simulink model "MCASSimulation__exp"  (R2022b)
settings: Solver=VariableStepAuto  StartTime=0.0  StopTime=350  RelTol=1e-3
model workspace (MAT data in the model file):
  ASd = 1
values from neighbouring files (symbols this model uses):
  sortedParams = table2struct(sortedT)    [RunSimulations.m]    (also in no_anomolies_run_handler.m)
libraries: slpidlib x12, simulink_extras x3
(part 3 of 4)

== matlab function MCASSimulation__exp/Human Pilot Simulator/Scripting Module/MATLAB Function Block ==
  data: JSBSim_data input; direct_to_JSBSim output; elevator_sp output; aileron_sp output; rudder_sp output; throttle_sp output; script input; horstab_sp output; script_parameters input; debug output
function [direct_to_JSBSim, elevator_sp, aileron_sp, rudder_sp, throttle_sp, horstab_sp, debug] = run(JSBSim_data, script, script_parameters)
%% Naming inputs from JSBSim
time_sec = JSBSim_data(1);
altitude_ASL_ft = JSBSim_data(2);
vert_speed_fps = JSBSim_data(3);
pitch_deg = JSBSim_data(4);
heading = JSBSim_data(5);
heading_rate_deg_sec = rad2deg(JSBSim_data(6));
roll_deg = JSBSim_data(7);
vc_kts = JSBSim_data(8);
engine_0_n1 = JSBSim_data(9);
engine_1_n1 = JSBSim_data(10);
elevator_cmd_norm = JSBSim_data(11);
stab_pos = JSBSim_data(12);
alpha = JSBSim_data(13);
mcas_is_firing = JSBSim_data(14);
mcas_cooldown_time = JSBSim_data(15);
mcas_trim_amount = JSBSim_data(16);
mcas_trim_rate = JSBSim_data(17);

mcas_duration_sec = mcas_trim_amount/mcas_trim_rate;

%% script parameters from workspace
persistent param_accel_start_spd;
persistent param_accel_end_spd;
persistent param_climb_starting_alt;
persistent param_climb_final_alt;
persistent param_desc_starting_alt;
persistent param_desc_final_alt;
persistent param_lvlturn_start_heading;
persistent param_lvlturn_turn_amount;
persistent param_climbturn_start_alt;
persistent param_climbturn_climb_amount;
persistent param_climbturn_start_heading;
persistent param_climbturn_turn_amount;
persistent param_holdpat_starting_heading;
persistent param_holdpat_leg_duration;
persistent param_takeoff_initial_climb_airspeed;
persistent param_takeoff_shallower_alt;
persistent param_takeoff_final_alt;
persistent param_takeoff_final_climb_airspeed;
persistent param_landing_desc_rate;
persistent param_landing_final_ref_airspeed;
persistent param_landing_start_alt;
persistent param_takeoffstall_target_pitch;
persistent param_takeoffstall_final_climb_airspeed;
persistent param_takeoffstall_pullup_time;
persistent param_pilot_reaction;

if isempty(param_accel_start_spd)
param_accel_start_spd = script_parameters(1);
param_accel_end_spd = script_parameters(2);
param_climb_starting_alt = script_parameters(3);
param_climb_final_alt = script_parameters(4);
param_desc_starting_alt = script_parameters(5);
param_desc_final_alt = script_parameters(6);
param_lvlturn_start_heading = script_parameters(7);
param_lvlturn_turn_amount = script_parameters(8);
param_climbturn_start_alt = script_parameters(9);
param_climbturn_climb_amount = script_parameters(10);
param_climbturn_start_heading = script_parameters(11);
param_climbturn_turn_amount = script_parameters(12);
param_holdpat_starting_heading = script_parameters(13);
param_holdpat_leg_duration = script_parameters(14);
param_takeoff_initial_climb_airspeed = script_parameters(15);
param_takeoff_shallower_alt = script_parameters(16);
param_takeoff_final_climb_airspeed = script_parameters(17);
param_takeoff_final_alt = script_parameters(18);
param_landing_desc_rate = script_parameters(19);
param_landing_final_ref_airspeed = script_parameters(20);
param_landing_start_alt = script_parameters(21);
param_takeoffstall_target_pitch = script_parameters(22);
param_takeoffstall_final_climb_airspeed = script_parameters(23);
param_takeoffstall_pullup_time = script_parameters(24);
param_pilot_reaction = script_parameters(25);
end

%% Naming controller modes
elevator_mode_off = 0;
elevator_mode_altitude = 1;
elevator_mode_vert_speed = 2;
elevator_mode_pitch = 3;
elevator_mode_airspeed = 4;
elevator_mode_direct = 5;
aileron_mode_off = 0;
aileron_mode_heading = 1;
aileron_mode_heading_rate = 2;
aileron_mode_roll = 3;
rudder_mode_off = 0;
rudder_mode_on = 1;
throttle_mode_off = 0;
throttle_mode_airspeed = 1;
throttle_mode_percent = 2;

%% Persistent variables
% Persistent variables retain their value between executions of the MATLAB function block, unlike 
% regular variables which are re-initialized each timestep of the simulation.
persistent engine_0_running;
persistent engine_1_running;
persistent landing_gear_cmd_norm;
persistent flap_cmd_norm;
persistent left_brake_cmd;
persistent right_brake_cmd;
persistent elevator_mode;
persistent ref_altitude;
persistent ref_vert_speed;
persistent ref_pitch;
persistent ref_direct;
persistent aileron_mode;
persistent ref_heading;
persistent ref_heading_rate;
persistent ref_roll;
persistent rudder_mode;
persistent ref_beta;
persistent throttle_mode;
persistent throttle_percent_norm;
persistent ref_vc;
persistent do_pilot_trim;
persistent trim_time_end;
persistent do_manual_trim;
persistent manual_trim_direction;
persistent manual_trim_time_end;
persistent lvlturn_turnto_heading;

% If a persistent variable is used only for a particular script, preface it's name with the name of the script it belongs to.
persistent level_turns_first_turn_done;

persistent climbturn_end_alt;
persistent climbturn_end_hdg;

persistent turn_then_descend_do_descent;

persistent holding_pattern_leg_timer;
persistent holding_pattern_outbound;
persistent holding_pattern_inbound;
persistent holding_pattern_inbound_heading;

persistent takeoff_step;
persistent takeoff_climb_vert_speed_fps;

persistent landing_step;

persistent takeoff_anomaly_stab_pos_start_anomaly;
persistent takeoff_anomaly_pullup_triggered;
persistent takeoff_anomaly_reacting_to_stall;
persistent takeoff_anomaly_last_mcas_turnon_time;
persistent takeoff_anomaly_retrim_start_time;

persistent takeoff_stall_pullup_triggered;
persistent takeoff_stall_reacting_to_stall;
persistent takeoff_stall_last_mcas_turnon_time;
persistent takeoff_stall_retrim_start_time;
persistent takeoff_stall_stab_pos_start_anomaly;
persistent reaction_time;


%% Scripts
switch script
    case "straight_and_level"
        if isempty(engine_0_running)
            engine_0_running = 1;
            engine_1_running = 1;
            landing_gear_cmd_norm = 0;
            flap_cmd_norm = 0;
            left_brake_cmd = 0;
            right_brake_cmd = 0;
            elevator_mode = elevator_mode_altitude;
            ref_altitude = 10000;
            ref_vert_speed = 10;
            ref_pitch = 15;
            ref_direct = 0;
            aileron_mode = aileron_mode_heading;
            ref_heading = 90;
            ref_heading_rate = 1;
            ref_roll = 15;
            rudder_mode = rudder_mode_on;
            ref_beta = 0;
            throttle_mode = throttle_mode_airspeed;
            throttle_percent_norm = 0;
            ref_vc = 240;
            do_pilot_trim = 0;  % pilot simulator will try to alleviate pressure from the elevator input
            trim_time_end = 0;
            do_manual_trim = 0;
            manual_trim_direction = 0;
            manual_trim_time_end = 0;
        end

    case "straight_and_level_accelerate"
        if isempty(engine_0_running)
            engine_0_running = 1;
            engine_1_running = 1;
            landing_gear_cmd_norm = 0;
            flap_cmd_norm = 0;
            left_brake_cmd = 0;
            right_brake_cmd = 0;
            elevator_mode = elevator_mode_altitude;
            ref_altitude = 10000;
            ref_vert_speed = 10;
            ref_pitch = 15;
            ref_direct = 0;
            aileron_mode = aileron_mode_heading;
            ref_heading = 90;
            ref_heading_rate = 1;
            ref_roll = 15;
            rudder_mode = rudder_mode_on;
            ref_beta = 0;
            throttle_mode = throttle_mode_airspeed;
            throttle_percent_norm = 0;
            ref_vc = param_accel_start_spd;
            do_pilot_trim = 0;  % pilot simulator will try to alleviate pressure from the elevator input
            trim_time_end = 0;
            do_manual_trim = 0;
            manual_trim_direction = 0;
            manual_trim_time_end = 0;
        end

        if time_sec > 15
            ref_vc = param_accel_end_spd;
        end

    case "straight_and_climb"
        if isempty(engine_0_running)
            engine_0_running = 1;
            engine_1_running = 1;
            landing_gear_cmd_norm = 0;
            flap_cmd_norm = 0;
            left_brake_cmd = 0;
            right_brake_cmd = 0;
            elevator_mode = elevator_mode_altitude;
            ref_altitude = param_climb_starting_alt;
            ref_vert_speed = 10;
            ref_pitch = 15;
            ref_direct = 0;
            aileron_mode = aileron_mode_heading;
            ref_heading = 90;
            ref_heading_rate = 1;
            ref_roll = 15;
            rudder_mode = rudder_mode_on;
            ref_beta = 0;
            throttle_mode = throttle_mode_airspeed;
            throttle_percent_norm = 0;
            ref_vc = 240;
            do_pilot_trim = 0;  % pilot simulator will try to alleviate pressure from the elevator input
            trim_time_end = 0;
            do_manual_trim = 0;
            manual_trim_direction = 0;
            manual_trim_time_end = 0;
        end

        if time_sec > 15
            ref_altitude = param_climb_final_alt;
        end

    case "straight_and_descend"
        if isempty(engine_0_running)
            engine_0_running = 1;
            engine_1_running = 1;
            landing_gear_cmd_norm = 0;
            flap_cmd_norm = 0;
            left_brake_cmd = 0;
            right_brake_cmd = 0;
            elevator_mode = elevator_mode_altitude;
            ref_altitude = param_desc_starting_alt;
            ref_vert_speed = 10;
            ref_pitch = 15;
            ref_direct = 0;
            aileron_mode = aileron_mode_heading;
            ref_heading = 90;
            ref_heading_rate = 1;
            ref_roll = 15;
            rudder_mode = rudder_mode_on;
            ref_beta = 0;
            throttle_mode = throttle_mode_airspeed;
            throttle_percent_norm = 0;
            ref_vc = 240;
            do_pilot_trim = 0;  % pilot simulator will try to alleviate pressure from the elevator input
            trim_time_end = 0;
            do_manual_trim = 0;
            manual_trim_direction = 0;
            manual_trim_time_end = 0;
        end

        if time_sec > 15
            ref_altitude = param_desc_final_alt;
        end

    case "level_turns"
        if isempty(engine_0_running)
            engine_0_running = 1;
            engine_1_running = 1;
            landing_gear_cmd_norm = 0;
            flap_cmd_norm = 0;
            left_brake_cmd = 0;
            right_brake_cmd = 0;
            elevator_mode = elevator_mode_altitude;
            ref_altitude = 10000;
            ref_vert_speed = 10;
            ref_pitch = 15;
            ref_direct = 0;
            aileron_mode = aileron_mode_heading;
            ref_heading = param_lvlturn_start_heading;
            ref_heading_rate = 1;
            ref_roll = 15;
            rudder_mode = rudder_mode_on;
            ref_beta = 0;
            throttle_mode = throttle_mode_airspeed;
            throttle_percent_norm = 0;
            ref_vc = 240;
            do_pilot_trim = 0;  % pilot simulator will try to alleviate pressure from the elevator input
            trim_time_end = 0;
            do_manual_trim = 0;
            manual_trim_direction = 0;
            manual_trim_time_end = 0;
        end
        
        if isempty(level_turns_first_turn_done) 
            level_turns_first_turn_done = 0;
            lvlturn_turnto_heading = param_lvlturn_start_heading + param_lvlturn_turn_amount;
        end

        if time_sec > 15 && ~level_turns_first_turn_done
            ref_heading = lvlturn_turnto_heading;
        end
        if heading > (lvlturn_turnto_heading-0.5) && heading < (lvlturn_turnto_heading+0.5)
            level_turns_first_turn_done = 1;
            ref_heading = param_lvlturn_start_heading;
        end

    case "climb_and_turn"
        if isempty(engine_0_running)
            engine_0_running = 1;
            engine_1_running = 1;
            landing_gear_cmd_norm = 0;
            flap_cmd_norm = 0;
            left_brake_cmd = 0;
            right_brake_cmd = 0;
            elevator_mode = elevator_mode_altitude;
            ref_altitude = param_climbturn_start_alt;
            ref_vert_speed = 10;
            ref_pitch = 15;
            ref_direct = 0;
            aileron_mode = aileron_mode_heading;
            ref_heading = param_climbturn_start_heading;
            ref_heading_rate = 1;
            ref_roll = 15;
            rudder_mode = rudder_mode_on;
            ref_beta = 0;
            throttle_mode = throttle_mode_airspeed;
            throttle_percent_norm = 0;
            ref_vc = 240;
            do_pilot_trim = 0;  % pilot simulator will try to alleviate pressure from the elevator input
            trim_time_end = 0;
            do_manual_trim = 0;
            manual_trim_direction = 0;
            manual_trim_time_end = 0;
        end
        if isempty(climbturn_end_alt)
            climbturn_end_alt = param_climbturn_start_alt + param_climbturn_climb_amount;
            climbturn_end_hdg = param_climbturn_start_heading + param_climbturn_turn_amount;
        end

        if time_sec > 15
            ref_altitude = climbturn_end_alt;
            ref_heading = climbturn_end_hdg;
        end

    case "descend_and_turn"
        if isempty(engine_0_running)
            engine_0_running = 1;
            engine_1_running = 1;
            landing_gear_cmd_norm = 0;
            flap_cmd_norm = 0;
            left_brake_cmd = 0;
            right_brake_cmd = 0;
            elevator_mode = elevator_mode_altitude;
            ref_altitude = 15000;
            ref_vert_speed = 10;
            ref_pitch = 15;
            ref_direct = 0;
            aileron_mode = aileron_mode_heading;
            ref_heading = 180;
            ref_heading_rate = 1;
            ref_roll = 15;
            rudder_mode = rudder_mode_on;
            ref_beta = 0;
            throttle_mode = throttle_mode_airspeed;
            throttle_percent_norm = 0;
            ref_vc = 240;
            do_pilot_trim = 0;  % pilot simulator will try to alleviate pressure from the elevator input
            trim_time_end = 0;
            do_manual_trim = 0;
            manual_trim_direction = 0;
            manual_trim_time_end = 0;
        end

        if time_sec > 15
            ref_altitude = 10000;
            ref_heading = 90;
        end

    case "turn_then_descend"
        if isempty(engine_0_running)
            engine_0_running = 1;
            engine_1_running = 1;
            landing_gear_cmd_norm = 0;
            flap_cmd_norm = 0;
            left_brake_cmd = 0;
            right_brake_cmd = 0;
            elevator_mode = elevator_mode_altitude;
            ref_altitude = 15000;
            ref_vert_speed = 10;
            ref_pitch = 15;
            ref_direct = 0;
            aileron_mode = aileron_mode_heading;
            ref_heading = 90;
            ref_heading_rate = 1;
            ref_roll = 15;
            rudder_mode = rudder_mode_on;
            ref_beta = 0;
            throttle_mode = throttle_mode_airspeed;
            throttle_percent_norm = 0;
            ref_vc = 240;
            do_pilot_trim = 0;  % pilot simulator will try to alleviate pressure from the elevator input
            trim_time_end = 0;
            do_manual_trim = 0;
            manual_trim_direction = 0;
            manual_trim_time_end = 0;
        end
        if isempty(turn_then_descend_do_descent)
            turn_then_descend_do_descent = 0;
        end

        if heading > 89.5 && heading < 90.5
            turn_then_descend_do_descent = 1;
        end

        if turn_then_descend_do_descent == 1
            ref_altitude = 12000;
        end

    case "holding_pattern"
        if isempty(engine_0_running)
            engine_0_running = 1;
            engine_1_running = 1;
            landing_gear_cmd_norm = 0;
            flap_cmd_norm = 0;
            left_brake_cmd = 0;
            right_brake_cmd = 0;
            elevator_mode = elevator_mode_altitude;
            ref_altitude = 10000;
            ref_vert_speed = 10;
            ref_pitch = 15;
            ref_direct = 0;
            aileron_mode = aileron_mode_heading;
            ref_heading = param_holdpat_starting_heading;
            ref_heading_rate = 1;
            ref_roll = -30; % negative = towards pilot's right
            rudder_mode = rudder_mode_on;
            ref_beta = 0;
            throttle_mode = throttle_mode_airspeed;
            throttle_percent_norm = 0;
            ref_vc = 240;
            do_pilot_trim = 0;  % pilot simulator will try to alleviate pressure from the elevator input
            trim_time_end = 0;
            do_manual_trim = 0;
            manual_trim_direction = 0;
            manual_trim_time_end = 0;
        end
        if isempty(holding_pattern_leg_timer)
            holding_pattern_leg_timer = 0;
        end
        if isempty(holding_pattern_outbound)
            holding_pattern_outbound = 0;
        end
        if isempty(holding_pattern_inbound)
            holding_pattern_inbound = 0;
        end
        if isempty(holding_pattern_inbound_heading)
            holding_pattern_inbound_heading = mod(param_holdpat_starting_heading + 180, 360);
        end

        % at heading 90
        % start timer
        if heading > (param_holdpat_starting_heading-0.5) && heading < (param_holdpat_starting_heading+0.5) && ~holding_pattern_outbound
            holding_pattern_leg_timer = time_sec;
            holding_pattern_outbound = 1;
        end

        % when timer reaches 60 seconds
        % switch aileron mode to bank 30
        if (time_sec - holding_pattern_leg_timer > param_holdpat_leg_duration) && holding_pattern_outbound
            aileron_mode = aileron_mode_roll;
        end

        % at heading 0
        % switch aileron mode to heading 270
        if heading > mod(param_holdpat_starting_heading-90.5, 360) && heading < mod(param_holdpat_starting_heading-89.5, 360) && holding_pattern_outbound
            aileron_mode = aileron_mode_heading;
            ref_heading = holding_pattern_inbound_heading;
            holding_pattern_outbound = 0;
        end

        % at heading 270
        % start timer
        if heading > (holding_pattern_inbound_heading-0.5) && heading < (holding_pattern_inbound_heading+0.5) && ~holding_pattern_inbound
            holding_pattern_leg_timer = time_sec;
            holding_pattern_inbound = 1;
        end

        % when timer reaches 60 seconds
        % switch aileron mode to bank 30
        if (time_sec - holding_pattern_leg_timer > param_holdpat_leg_duration) && holding_pattern_inbound
            aileron_mode = aileron_mode_roll;
        end

        % at heading 180
        % switch aileron mode to heading 90
        if heading > mod(param_holdpat_starting_heading+89.5, 360) && heading < mod(param_holdpat_starting_heading+90.5, 360) && holding_pattern_inbound
            aileron_mode = aileron_mode_heading;
            ref_heading = param_holdpat_starting_heading;
            holding_pattern_inbound = 0;
        end

    case "takeoff"
        if isempty(engine_0_running)
            engine_0_running = 1;
            engine_1_running = 1;
            landing_gear_cmd_norm = 1;
            flap_cmd_norm = 0.375;
            left_brake_cmd = 0;
            right_brake_cmd = 0;
            elevator_mode = elevator_mode_off;
            ref_altitude = 1000;
            ref_vert_speed = 10;
            ref_pitch = 30;
            ref_direct = 0;
            aileron_mode = aileron_mode_heading;
            ref_heading = 90;
            ref_heading_rate = 1;
            ref_roll = 15;
            rudder_mode = rudder_mode_on;
            ref_beta = 0;
            throttle_mode = throttle_mode_percent;
            throttle_percent_norm = 0;
            ref_vc = 0;
            do_pilot_trim = 0;  % pilot simulator will try to alleviate pressure from the elevator input
            trim_time_end = 0;
            do_manual_trim = 0;
            manual_trim_direction = 1;
            manual_trim_time_end = 0;
        end
        if isempty(takeoff_step)
            takeoff_step = 0;   % for ensuring each step only executes once
            takeoff_climb_vert_speed_fps = 0;
        end

        if time_sec < trim_time_end
            do_pilot_trim = 1;
        end
        if time_sec > trim_time_end
            do_pilot_trim = 0;
        end

        if time_sec > 15 && takeoff_step == 0
            throttle_percent_norm = 0.5;
            takeoff_step = takeoff_step + 1;
        end

        if engine_0_n1 > 40 && engine_1_n1 > 40 && takeoff_step == 1
            throttle_percent_norm = 0.95;
            takeoff_step = takeoff_step + 1;
        end

        if vc_kts > 150 && takeoff_step == 2    % Plane will not lift off until about 150
            elevator_mode = elevator_mode_pitch;
            ref_pitch = 10;
            takeoff_step = takeoff_step + 1;
        end

        if vc_kts > (param_takeoff_initial_climb_airspeed-10) && altitude_ASL_ft > 50 && takeoff_step == 3
            landing_gear_cmd_norm = 0;
            elevator_mode = elevator_mode_airspeed;
            ref_vc = param_takeoff_initial_climb_airspeed;
            takeoff_step = takeoff_step + 1;
        end

        if altitude_ASL_ft > 500 && takeoff_step == 4
%             trim_time_end = time_sec + 5;
            takeoff_step = takeoff_step + 1;
        end

        % 1600 ft chosen to match Lion Air crash data
        if altitude_ASL_ft > param_takeoff_shallower_alt && takeoff_step == 5
            takeoff_climb_vert_speed_fps = vert_speed_fps;
            elevator_mode = elevator_mode_vert_speed;
            ref_vert_speed = takeoff_climb_vert_speed_fps / 2;

            throttle_mode = throttle_mode_airspeed;
            ref_vc = param_takeoff_final_climb_airspeed;

            takeoff_step = takeoff_step + 1;
        end

        if altitude_ASL_ft > (param_takeoff_shallower_alt+500) && takeoff_step == 6
            trim_time_end = time_sec + 5;
            takeoff_step = takeoff_step + 1;
        end

        if vc_kts > 190
            flap_cmd_norm = 0.125;
        end

        if vc_kts > 210
            flap_cmd_norm = 0;
        end

        if altitude_ASL_ft > (param_takeoff_final_alt-500) && takeoff_step == 7     % at this point, takeoff and initial climb procedures are over, and we climb to cruise at arbitrary 15k feet.
            elevator_mode = elevator_mode_altitude;
            ref_altitude = param_takeoff_final_alt;
            takeoff_step = takeoff_step + 1;
        end

    case "landing"
       if isempty(engine_0_running)
            engine_0_running = 1;
            engine_1_running = 1;
            landing_gear_cmd_norm = 1;
            flap_cmd_norm = 0.375;
            left_brake_cmd = 0;
            right_brake_cmd = 0;
            elevator_mode = elevator_mode_altitude;
            ref_altitude = param_landing_start_alt;
            ref_vert_speed = param_landing_desc_rate;    % -700 fpm = -11.67 fps
            ref_pitch = 30;
            ref_direct = 0;
            aileron_mode = aileron_mode_heading;
            ref_heading = 90;
            ref_heading_rate = 1;
            ref_roll = 15;
            rudder_mode = rudder_mode_on;
            ref_beta = 0;
            throttle_mode = throttle_mode_airspeed;
            throttle_percent_norm = 0;
            ref_vc = 200;
            do_pilot_trim = 0;  % pilot simulator will try to alleviate pressure from the elevator input
            trim_time_end = 0;
            do_manual_trim = 0;
            manual_trim_direction = 0;
            manual_trim_time_end = 0;
       end
       if isempty(landing_step)
            landing_step = 0;   % for ensuring each step only executes once
       end

       if time_sec > 15 && landing_step == 0 
            ref_vc = param_landing_final_ref_airspeed;
            landing_step = landing_step + 1;
       end

       if vc_kts < 170 && landing_step == 1
            flap_cmd_norm = 0.5;
            landing_step = landing_step + 1;
       end

       if vc_kts < (param_landing_final_ref_airspeed+15) && landing_step == 2
           elevator_mode = elevator_mode_vert_speed;
           landing_step = landing_step + 1;
       end

       if vc_kts < 150 && landing_step == 3
           flap_cmd_norm = 0.625;
           landing_step = landing_step + 1;
       end

       if vc_kts < 140 && landing_step == 4
           flap_cmd_norm = 0.875;
           landing_step = landing_step + 1;
       end

    case "takeoff_stall_perfect_pilot"
       if isempty(engine_0_running)
            engine_0_running = 1;
            engine_1_running = 1;
            landing_gear_cmd_norm = 1;
            flap_cmd_norm = 0.375;
            left_brake_cmd = 0;
            right_brake_cmd = 0;
            elevator_mode = elevator_mode_off;
            ref_altitude = 1000;
            ref_vert_speed = 10;
            ref_pitch = 30;
            ref_direct = 0;
            aileron_mode = aileron_mode_heading;
            ref_heading = 90;
            ref_heading_rate = 1;
            ref_roll = 15;
            rudder_mode = rudder_mode_on;
            ref_beta = 0;
            throttle_mode = throttle_mode_percent;
            throttle_percent_norm = 0;
            ref_vc = 0;
            do_pilot_trim = 0;  % pilot simulator will try to alleviate pressure from the elevator input
            trim_time_end = 0;
            do_manual_trim = 0;
            manual_trim_direction = 0;
            manual_trim_time_end = 0;
        end
        if isempty(takeoff_step)
            takeoff_step = 0;   % for ensuring each step only executes once
            takeoff_climb_vert_speed_fps = 0;
        end
        if isempty(takeoff_stall_pullup_triggered)
            takeoff_stall_pullup_triggered = 0;
        end

        if time_sec > param_takeoffstall_pullup_time && ~takeoff_stall_pullup_triggered
            takeoff_stall_pullup_triggered = 1;
            elevator_mode = elevator_mode_pitch;
            ref_pitch = param_takeoffstall_target_pitch;
        end

        if alpha > 12 && takeoff_stall_pullup_triggered && takeoff_step ~= -1
            % this is where pilot begins to take action for stall
            % avoidance and recovery
            takeoff_step = -1;
            elevator_mode = elevator_mode_direct;   % aggressive nose-down to avoid immediate stall
            ref_direct = 0.6;
            throttle_mode = throttle_mode_percent;
            throttle_percent_norm = 1;
        end

        if pitch_deg < 5 && takeoff_step == -1
            takeoff_step = -2;
            elevator_mode = elevator_mode_pitch;
            ref_pitch = -4;
        end

        if vc_kts > 220 && takeoff_step == -2
            takeoff_step = 5;

            elevator_mode = elevator_mode_vert_speed;
            ref_vert_speed = takeoff_climb_vert_speed_fps / 2;  % doesn't exist if stall is initiated BEFORE the 'shallowing' step of takeoff (step 4)

            throttle_mode = throttle_mode_airspeed;
            ref_vc = param_takeoffstall_final_climb_airspeed;
        end

        if time_sec > 15 && takeoff_step == 0
            throttle_percent_norm = 0.5;
            takeoff_step = takeoff_step + 1;
        end

        if engine_0_n1 > 40 && engine_1_n1 > 40 && takeoff_step == 1
            throttle_percent_norm = 0.95;
            takeoff_step = takeoff_step + 1;
        end

        if vc_kts > 150 && takeoff_step == 2
            elevator_mode = elevator_mode_pitch;
            ref_pitch = 10;
            takeoff_step = takeoff_step + 1;
        end

        if vc_kts > 170 && altitude_ASL_ft > 50 && takeoff_step == 3
            landing_gear_cmd_norm = 0;
            elevator_mode = elevator_mode_airspeed;
            ref_vc = 170;
            takeoff_step = takeoff_step + 1;
        end

        % 1600 ft chosen to match Lion Air crash data
        if altitude_ASL_ft > 1600 && takeoff_step == 4
            takeoff_climb_vert_speed_fps = vert_speed_fps;
            elevator_mode = elevator_mode_vert_speed;
            ref_vert_speed = takeoff_climb_vert_speed_fps / 2;

            throttle_mode = throttle_mode_airspeed;
            ref_vc = param_takeoffstall_final_climb_airspeed;

            takeoff_step = takeoff_step + 1;
        end

        if vc_kts > 190 && takeoff_step == 5
            flap_cmd_norm = 0.125;
            takeoff_step = takeoff_step + 1;
        end

        if vc_kts > 210 && takeoff_step == 6
            flap_cmd_norm = 0;
            takeoff_step = takeoff_step + 1;
        end

    case "takeoff_stall_pilot_reaction_delay"
       if isempty(engine_0_running)
            engine_0_running = 1;
            engine_1_running = 1;
            landing_gear_cmd_norm = 1;
            flap_cmd_norm = 0.375;
            left_brake_cmd = 0;
            right_brake_cmd = 0;
            elevator_mode = elevator_mode_off;
            ref_altitude = 1000;
            ref_vert_speed = 10;
            ref_pitch = 30;
            ref_direct = 0;
            aileron_mode = aileron_mode_heading;
            ref_heading = 90;
            ref_heading_rate = 1;
            ref_roll = 15;
            rudder_mode = rudder_mode_on;
            ref_beta = 0;
            throttle_mode = throttle_mode_percent;
            throttle_percent_norm = 0;
            ref_vc = 0;
            do_pilot_trim = 0;  % pilot simulator will try to alleviate pressure from the elevator input
            trim_time_end = 0;
            do_manual_trim = 0;
            manual_trim_direction = 0;
            manual_trim_time_end = 0;
        end
        if isempty(takeoff_step)
            takeoff_step = 0;   % for ensuring each step only executes once
            takeoff_climb_vert_speed_fps = 0;
        end
        if isempty(takeoff_stall_pullup_triggered)
            takeoff_stall_pullup_triggered = 0;
        end
        if isempty(takeoff_stall_reacting_to_stall)
            takeoff_stall_reacting_to_stall = 0;
        end
        if isempty(takeoff_stall_last_mcas_turnon_time)
            takeoff_stall_last_mcas_turnon_time = -999;  % setting to 0 causes issues at start
        end
        if isempty(takeoff_stall_retrim_start_time)
            takeoff_stall_retrim_start_time = -999;  % setting to 0 causes issues at start
        end
        if isempty(takeoff_stall_stab_pos_start_anomaly)
            takeoff_stall_stab_pos_start_anomaly = 0;
        end

        if time_sec > takeoff_stall_retrim_start_time && time_sec < trim_time_end
            do_pilot_trim = 1;
        end
        if time_sec > trim_time_end
            do_pilot_trim = 0;
        end

        if mcas_is_firing && (time_sec-takeoff_stall_last_mcas_turnon_time) > mcas_duration_sec
            takeoff_stall_last_mcas_turnon_time = time_sec;
        end

        % stop trimming if MCAS fires (trim wheel is yanked from pilot)
        if (time_sec-takeoff_stall_last_mcas_turnon_time) > 0 && (time_sec-takeoff_stall_last_mcas_turnon_time) < 1
            trim_time_end = 0;
        end
        
        if time_sec > param_takeoffstall_pullup_time && ~takeoff_stall_pullup_triggered
            takeoff_stall_pullup_triggered = 1;
            elevator_mode = elevator_mode_pitch;
            ref_pitch = param_takeoffstall_target_pitch;
        end

        % these cause additional stall maneuvers
        %if time_sec > 200 && time_sec < 201
        %    takeoff_stall_pullup_triggered = 0;
        %end
        %if time_sec > 300 && time_sec < 301
        %    takeoff_stall_pullup_triggered = 0;
        %end

        % If AoA<10 when MCAS triggers, fight against MCAS and trim.
        % This is the case where MCAS is 'errant'.
        if (time_sec-takeoff_stall_last_mcas_turnon_time) > 0 && (time_sec-takeoff_stall_last_mcas_turnon_time) < 0.1
            takeoff_stall_retrim_start_time = time_sec + param_pilot_reaction + mcas_duration_sec;
        end

        if (time_sec-takeoff_stall_retrim_start_time) > 0 && (time_sec-takeoff_stall_retrim_start_time) < 0.1 && ~takeoff_stall_reacting_to_stall
            trim_time_end = time_sec + 2.5/(3.5/18);
        end

        % If AoA>10 when MCAS triggers, do stall recovery after reaction delay.
        % This is the case where MCAS is 'correct'.
        if (time_sec-takeoff_stall_last_mcas_turnon_time) > param_pilot_reaction && (time_sec-takeoff_stall_last_mcas_turnon_time) < param_pilot_reaction+0.1 && ~takeoff_stall_reacting_to_stall && alpha > 10
            takeoff_step = -1;
            takeoff_stall_reacting_to_stall = 1;
            elevator_mode = elevator_mode_direct;   % aggressive nose-down to avoid immediate stall
            ref_direct = 0.6;
            throttle_mode = throttle_mode_percent;
            throttle_percent_norm = 1;
        end

        if pitch_deg < 5 && takeoff_step == -1
            takeoff_step = -2;
            elevator_mode = elevator_mode_pitch;
            ref_pitch = -10;
        end
        
        % resume normal flight
        if vc_kts > 220 && takeoff_step == -2 
            takeoff_step = 5;
            takeoff_stall_reacting_to_stall = 0;
            elevator_mode = elevator_mode_vert_speed;
            ref_vert_speed = takeoff_climb_vert_speed_fps / 2;  % doesn't exist if stall is initiated BEFORE the 'shallowing' step of takeoff (step 4)
            throttle_mode = throttle_mode_airspeed;
            ref_vc = param_takeoffstall_final_climb_airspeed;
            trim_time_end = time_sec + mcas_cooldown_time;
        end

        if time_sec > 15 && takeoff_step == 0
            throttle_percent_norm = 0.5;
            takeoff_step = takeoff_step + 1;
        end

        if engine_0_n1 > 40 && engine_1_n1 > 40 && takeoff_step == 1
            throttle_percent_norm = 0.95;
            takeoff_step = takeoff_step + 1;
        end

        if vc_kts > 150 && takeoff_step == 2
            elevator_mode = elevator_mode_pitch;
            ref_pitch = 10;
            takeoff_step = takeoff_step + 1;
        end

        if vc_kts > 170 && altitude_ASL_ft > 50 && takeoff_step == 3
            landing_gear_cmd_norm = 0;
            elevator_mode = elevator_mode_airspeed;
            ref_vc = 170;
            takeoff_step = takeoff_step + 1;
        end

        % 1600 ft chosen to match Lion Air crash data
        if altitude_ASL_ft > 1600 && takeoff_step == 4
            takeoff_climb_vert_speed_fps = vert_speed_fps;
            elevator_mode = elevator_mode_vert_speed;
            ref_vert_speed = takeoff_climb_vert_speed_fps / 2;

            throttle_mode = throttle_mode_airspeed;
            ref_vc = param_takeoffstall_final_climb_airspeed;

            takeoff_step = takeoff_step + 1;
        end

        if vc_kts > 190 && takeoff_step == 5
            flap_cmd_norm = 0.125;
            takeoff_step = takeoff_step + 1;
        end

        if vc_kts > 210 && takeoff_step == 6
            flap_cmd_norm = 0;
            takeoff_step = takeoff_step + 1;
        end

        if (time_sec-takeoff_stall_retrim_start_time) > 0 && (time_sec-takeoff_stall_retrim_start_time) < 0.1 && takeoff_step == 7
            elevator_mode = elevator_mode_direct;
            ref_direct = elevator_cmd_norm;
            takeoff_stall_stab_pos_start_anomaly = stab_pos;
            
            takeoff_step = takeoff_step + 1;
        end

        if (time_sec-takeoff_stall_retrim_start_time) > param_pilot_reaction && (time_sec-takeoff_stall_retrim_start_time) < param_pilot_reaction+0.1 && takeoff_step == 8

            if takeoff_stall_stab_pos_start_anomaly ~= stab_pos  
                elevator_mode = elevator_mode_direct;
                ref_direct = -0.1;
            else
                elevator_mode = elevator_mode_vert_speed;
                ref_vert_speed = takeoff_climb_vert_speed_fps / 2;
            end

            takeoff_step = takeoff_step + 1;
        end

        if time_sec > 100 + param_pilot_reaction + 10 && takeoff_step == 10
           % if takeoff_anomaly_stab_pos_start_anomaly ~= stab_pos  
           %     elevator_mode = elevator_mode_direct;
           %     ref_direct = -0.15;
           % else
           %     elevator_mode = elevator_mode_vert_speed;
           %     ref_vert_speed = takeoff_climb_vert_speed_fps / 2;
           % end

            takeoff_step = takeoff_step + 1;
        end

    case "takeoff_anomaly"
        if isempty(engine_0_running)
            engine_0_running = 1;
            engine_1_running = 1;
            landing_gear_cmd_norm = 1;
            flap_cmd_norm = 0.375;
            left_brake_cmd = 0;
            right_brake_cmd = 0;
            elevator_mode = elevator_mode_off;
            ref_altitude = 1000;
            ref_vert_speed = 10;
            ref_pitch = 30;
            ref_direct = 0;
            aileron_mode = aileron_mode_heading;
            ref_heading = 90;
            ref_heading_rate = 1;
            ref_roll = 15;
            rudder_mode = rudder_mode_on;
            ref_beta = 0;
            throttle_mode = throttle_mode_percent;
            throttle_percent_norm = 0;
            ref_vc = 0;
            do_pilot_trim = 0;  % pilot simulator will try to alleviate pressure from the elevator input
            trim_time_end = 0;
            do_manual_trim = 0;
            manual_trim_direction = 1;
            manual_trim_time_end = 0;
        end
        if isempty(takeoff_step)
            takeoff_step = 0;   % for ensuring each step only executes once
            takeoff_climb_vert_speed_fps = 0;
        end
        if isempty(takeoff_anomaly_stab_pos_start_anomaly)
            takeoff_anomaly_stab_pos_start_anomaly = 0;
        end
        if isempty(takeoff_anomaly_pullup_triggered)
            takeoff_anomaly_pullup_triggered = 0;
        end
        if isempty(takeoff_anomaly_reacting_to_stall)
            takeoff_anomaly_reacting_to_stall = 0;
        end
        if isempty(takeoff_anomaly_last_mcas_turnon_time)
            takeoff_anomaly_last_mcas_turnon_time = -999;  % setting to 0 causes issues at start
        end
        if isempty(takeoff_anomaly_retrim_start_time)
            takeoff_anomaly_retrim_start_time = -999;  % setting to 0 causes issues at start
        end

        if time_sec < trim_time_end
            do_manual_trim = 1;
        end
        if time_sec > trim_time_end
            do_manual_trim = 0;
        end

        if mcas_is_firing && (time_sec-takeoff_anomaly_last_mcas_turnon_time) > mcas_duration_sec
            takeoff_anomaly_last_mcas_turnon_time = time_sec;
        end

        % stop trimming if MCAS fires (trim wheel is yanked from pilot)
        if (time_sec-takeoff_anomaly_last_mcas_turnon_time) > 0 && (time_sec-takeoff_anomaly_last_mcas_turnon_time) < 1
            trim_time_end = 0;
        end

        % these cause additional stall maneuvers
        %if time_sec > 200 && time_sec < 201
        %    takeoff_stall_pullup_triggered = 0;
        %end
        %if time_sec > 300 && time_sec < 301
        %    takeoff_stall_pullup_triggered = 0;
        %end

        % If AoA<10 when MCAS triggers, fight against MCAS and trim.
        % This is the case where MCAS is 'errant'.
        if (time_sec-takeoff_anomaly_last_mcas_turnon_time) > param_pilot_reaction && (time_sec-takeoff_anomaly_last_mcas_turnon_time) < param_pilot_reaction+0.1
            takeoff_anomaly_retrim_start_time = time_sec + mcas_duration_sec;
        end

        if (time_sec-takeoff_anomaly_retrim_start_time) > param_pilot_reaction && (time_sec-takeoff_anomaly_last_mcas_turnon_time) < param_pilot_reaction+0.1 && ~takeoff_anomaly_reacting_to_stall
            trim_time_end = time_sec + mcas_cooldown_time;
        end

        % If AoA>10 when MCAS triggers, do stall recovery after reaction delay.
        % This is the case where MCAS is 'correct'.
        %if (time_sec-takeoff_anomaly_last_mcas_turnon_time) > param_pilot_reaction && (time_sec-takeoff_anomaly_last_mcas_turnon_time) < param_pilot_reaction+0.1 && ~takeoff_anomaly_reacting_to_stall && alpha > 10
        %    takeoff_step = -1;
        %    takeoff_anomaly_reacting_to_stall = 1;
        %    elevator_mode = elevator_mode_direct;   % aggressive nose-down to avoid immediate stall
        %    ref_direct = 0.6;
        %    throttle_mode = throttle_mode_percent;
        %    throttle_percent_norm = 1;
        %end

        %if pitch_deg < 5 && takeoff_step == -1
        %    takeoff_step = -2;
        %    elevator_mode = elevator_mode_pitch;
        %    ref_pitch = -10;
        %end
        
        % resume normal flight
        %if vc_kts > 220 && takeoff_step == -2 
        %    takeoff_step = 5;
        %    takeoff_anomaly_reacting_to_stall = 0;
        %    elevator_mode = elevator_mode_vert_speed;
        %    ref_vert_speed = takeoff_climb_vert_speed_fps / 2;  % doesn't exist if stall is initiated BEFORE the 'shallowing' step of takeoff (step 4)
        %    throttle_mode = throttle_mode_airspeed;
        %    ref_vc = param_takeoffstall_final_climb_airspeed;
        %    trim_time_end = time_sec + mcas_cooldown_time;
        %end

        if time_sec > 15 && takeoff_step == 0
            throttle_percent_norm = 0.5;
            takeoff_step = takeoff_step + 1;
        end

        if engine_0_n1 > 40 && engine_1_n1 > 40 && takeoff_step == 1
            throttle_percent_norm = 0.95;
            takeoff_step = takeoff_step + 1;
        end

        if vc_kts > 150 && takeoff_step == 2
            elevator_mode = elevator_mode_pitch;
            ref_pitch = 3;
            takeoff_step = takeoff_step + 1;
        end

        if vc_kts > 170 && altitude_ASL_ft > 50 && takeoff_step == 3
            landing_gear_cmd_norm = 0;
            elevator_mode = elevator_mode_airspeed;
            ref_vc = 170;
            takeoff_step = takeoff_step + 1;
        end

        if altitude_ASL_ft > 500 && takeoff_step == 4
            trim_time_end = time_sec + 5;
            takeoff_step = takeoff_step + 1;
        end

        % 1600 ft chosen to match Lion Air crash data
        if altitude_ASL_ft > 1600 && takeoff_step == 5
            takeoff_climb_vert_speed_fps = vert_speed_fps;
            elevator_mode = elevator_mode_vert_speed;
            ref_vert_speed = takeoff_climb_vert_speed_fps / 2;

            throttle_mode = throttle_mode_airspeed;
            ref_vc = 250;

            takeoff_step = takeoff_step + 1;
        end

        if altitude_ASL_ft > 2100 && takeoff_step == 6
            trim_time_end = time_sec + 5;
            takeoff_step = takeoff_step + 1;
        end

        if vc_kts > 190 && takeoff_step == 7
            flap_cmd_norm = 0.125;
            takeoff_step = takeoff_step + 1;
        end

        if time_sec > 100 && takeoff_step == 8
            elevator_mode = elevator_mode_direct;
            ref_direct = elevator_cmd_norm;
            takeoff_anomaly_stab_pos_start_anomaly = stab_pos;
            takeoff_step = takeoff_step + 1;
        end

        if time_sec > 100 + param_pilot_reaction && takeoff_step == 9
            if takeoff_anomaly_stab_pos_start_anomaly ~= stab_pos  
                elevator_mode = elevator_mode_direct;
                ref_direct = -0.3;
            else
                elevator_mode = elevator_mode_vert_speed;
                ref_vert_speed = takeoff_climb_vert_speed_fps / 2;
            end

            takeoff_step = takeoff_step + 1;
        end

        if time_sec > 100 + param_pilot_reaction + 10 && takeoff_step == 10
            if takeoff_anomaly_stab_pos_start_anomaly ~= stab_pos  
                elevator_mode = elevator_mode_direct;
                ref_direct = -0.15;
            else
                elevator_mode = elevator_mode_vert_speed;
                ref_vert_speed = takeoff_climb_vert_speed_fps / 2;
            end

            takeoff_step = takeoff_step + 1;
        end

    case "takeoff_JT610_no_intervention"
        if isempty(engine_0_running)
            engine_0_running = 1;
            engine_1_running = 1;
            landing_gear_cmd_norm = 1;
            flap_cmd_norm = 0.375;
            left_brake_cmd = 0;
            right_brake_cmd = 0;
            elevator_mode = elevator_mode_off;
            ref_altitude = 1000;
            ref_vert_speed = 10;
            ref_pitch = 30;
            ref_direct = 0;
            aileron_mode = aileron_mode_heading;
            ref_heading = 90;
            ref_heading_rate = 1;
            ref_roll = 15;
            rudder_mode = rudder_mode_on;
            ref_beta = 0;
            throttle_mode = throttle_mode_percent;
            throttle_percent_norm = 0;
            ref_vc = 0;
            do_pilot_trim = 0;  % pilot simulator will try to alleviate pressure from the elevator input
            trim_time_end = 0;
            do_manual_trim = 0;
            manual_trim_direction = 1;
            manual_trim_time_end = 0;
        end
        if isempty(takeoff_step)
            takeoff_step = 0;   % for ensuring each step only executes once
            takeoff_climb_vert_speed_fps = 0;
        end

        if time_sec < trim_time_end
            do_pilot_trim = 1;
        end
        if time_sec > trim_time_end
            do_pilot_trim = 0;
        end

        if time_sec < manual_trim_time_end
            do_manual_trim = 1;
        end
        if time_sec > manual_trim_time_end
            do_manual_trim = 0;
        end

        if time_sec > 15 && takeoff_step == 0
            throttle_percent_norm = 0.375;
            takeoff_step = takeoff_step + 1;
        end

        if engine_0_n1 > 35 && engine_1_n1 > 35 && takeoff_step == 1
            throttle_percent_norm = 0.75;
            takeoff_step = takeoff_step + 1;
        end

        if vc_kts > 200 && takeoff_step == 2
            elevator_mode = elevator_mode_pitch;
            ref_pitch = 2.9;
            takeoff_step = takeoff_step + 1;
        end

        if vc_kts > 210 && altitude_ASL_ft > 40 && takeoff_step == 3
            landing_gear_cmd_norm = 0;
            takeoff_step = takeoff_step + 1;
        end
 
         if altitude_ASL_ft > 500 && takeoff_step == 4
             trim_time_end = time_sec + 8;
             elevator_mode = elevator_mode_pitch;
             ref_pitch = 2;
             takeoff_step = takeoff_step + 1;
         end

         if altitude_ASL_ft > 1430 && takeoff_step == 5
 
             elevator_mode = elevator_mode_pitch;
             ref_pitch = -0.3;
             flap_cmd_norm = 0.25;
 
             takeoff_step = takeoff_step + 1;
         end
 
         if altitude_ASL_ft > 1950 && takeoff_step == 6
             elevator_mode = elevator_mode_pitch;
             ref_pitch = 3;
 
             takeoff_step = takeoff_step + 1;
         end

        if time_sec > 156 && takeoff_step == 7
            elevator_mode = elevator_mode_pitch;
            ref_pitch = 1.3;
            flap_cmd_norm = 0;

            takeoff_step = takeoff_step + 1;
        end

        if time_sec > 162.5 && takeoff_step == 8
            elevator_mode = elevator_mode_off;

            takeoff_step = takeoff_step + 1;
        end

%         if time_sec > 165.85 && takeoff_step == 9
% 
%             flap_cmd_norm = 0.25;
% 
%             takeoff_step = takeoff_step + 1;
%         end
% 
%         if time_sec > 173.6 && takeoff_step == 10
%             manual_trim_time_end = time_sec + 3.5;
%             manual_trim_direction = 1;
% 
%             takeoff_step = takeoff_step + 1;
%         end
% 
%         if time_sec > 187.1 && takeoff_step == 11
%           
%             flap_cmd_norm = 1;
%             elevator_mode = elevator_mode_pitch;
%             ref_pitch = -8.1;
% 
%             takeoff_step = takeoff_step + 1;
%         end
% 
%         if time_sec > 187.5 && takeoff_step == 12
%             manual_trim_time_end = time_sec + 3;
%             manual_trim_direction = 1;
% 
%             takeoff_step = takeoff_step + 1;
%         end

    case "takeoff_JT610"
        if isempty(engine_0_running)
            engine_0_running = 1;
            engine_1_running = 1;
            landing_gear_cmd_norm = 1;
            flap_cmd_norm = 0.375;
            left_brake_cmd = 0;
            right_brake_cmd = 0;
            elevator_mode = elevator_mode_off;
            ref_altitude = 1000;
            ref_vert_speed = 10;
            ref_pitch = 30;
            ref_direct = 0;
            aileron_mode = aileron_mode_heading;
            ref_heading = 90;
            ref_heading_rate = 1;
            ref_roll = 15;
            rudder_mode = rudder_mode_on;
            ref_beta = 0;
            throttle_mode = throttle_mode_percent;
            throttle_percent_norm = 0;
            ref_vc = 0;
            do_pilot_trim = 0;  % pilot simulator will try to alleviate pressure from the elevator input
            trim_time_end = 0;
            do_manual_trim = 0;
            manual_trim_direction = 0;
            manual_trim_time_end = 0;
        end
        if isempty(takeoff_step)
            takeoff_step = 0;   % for ensuring each step only executes once
            takeoff_climb_vert_speed_fps = 0;
        end

        if time_sec < trim_time_end
            do_pilot_trim = 1;
        end
        if time_sec > trim_time_end
            do_pilot_trim = 0;
        end

        if time_sec < manual_trim_time_end
            do_manual_trim = 1;
        end
        if time_sec > manual_trim_time_end
            do_manual_trim = 0;
        end

        if time_sec > 15 && takeoff_step == 0
            throttle_percent_norm = 0.375;
            takeoff_step = takeoff_step + 1;
        end

        if engine_0_n1 > 35 && engine_1_n1 > 35 && takeoff_step == 1
            throttle_percent_norm = 0.75;
            takeoff_step = takeoff_step + 1;
        end

        if vc_kts > 200 && takeoff_step == 2
            elevator_mode = elevator_mode_pitch;
            ref_pitch = 2.9;
            takeoff_step = takeoff_step + 1;
        end

        if vc_kts > 210 && altitude_ASL_ft > 40 && takeoff_step == 3
            landing_gear_cmd_norm = 0;
            takeoff_step = takeoff_step + 1;
        end
 
         if altitude_ASL_ft > 500 && takeoff_step == 4
             trim_time_end = time_sec + 8;
             elevator_mode = elevator_mode_pitch;
             ref_pitch = 2;
             takeoff_step = takeoff_step + 1;
         end

         if altitude_ASL_ft > 1430 && takeoff_step == 5
 
             elevator_mode = elevator_mode_pitch;
             ref_pitch = -0.3;
             flap_cmd_norm = 0.25;
 
             takeoff_step = takeoff_step + 1;
         end
 
         if altitude_ASL_ft > 1950 && takeoff_step == 6
             elevator_mode = elevator_mode_pitch;
             ref_pitch = 3;
 
             takeoff_step = takeoff_step + 1;
         end

        if time_sec > 156 && takeoff_step == 7
            elevator_mode = elevator_mode_pitch;
            ref_pitch = 1.3;
            flap_cmd_norm = 0;

            takeoff_step = takeoff_step + 1;
        end

        if time_sec > 162.5 && takeoff_step == 8
            elevator_mode = elevator_mode_off;

            takeoff_step = takeoff_step + 1;
        end

        if time_sec > 165.85 && takeoff_step == 9

            flap_cmd_norm = 0.25;

            takeoff_step = takeoff_step + 1;
        end

        if time_sec > 173.6 && takeoff_step == 10
            manual_trim_time_end = time_sec + 3.5;
            manual_trim_direction = 1;

            takeoff_step = takeoff_step + 1;
        end

        if time_sec > 187.1 && takeoff_step == 11
          
            flap_cmd_norm = 1;
            elevator_mode = elevator_mode_pitch;
            ref_pitch = -8.1;

            takeoff_step = takeoff_step + 1;
        end

        if time_sec > 187.5 && takeoff_step == 12
            manual_trim_time_end = time_sec + 3;
            manual_trim_direction = 1;

            takeoff_step = takeoff_step + 1;
        end

        if time_sec > 200 && takeoff_step == 13
            trim_time_end = time_sec + 3;

            takeoff_step = takeoff_step + 1;
        end

        if time_sec > 203 && takeoff_step == 14
            ref_pitch = -3.6;

            takeoff_step = takeoff_step + 1;
        end

        if time_sec > 250 && takeoff_step == 15
            manual_trim_time_end = time_sec + 1.25;
            manual_trim_direction = -1;

            ref_pitch = -3;

            takeoff_step = takeoff_step + 1;
        end

        if time_sec > 275 && takeoff_step == 16
            manual_trim_time_end = time_sec + 2.25;
            manual_trim_direction = 1;

            elevator_mode = elevator_mode_altitude;
            ref_altitude = 5350;

            takeoff_step = takeoff_step + 1;
        end

        if time_sec > 300 && takeoff_step == 17
            elevator_mode = elevator_mode_pitch;
            ref_pitch = -4;

            flap_cmd_norm = 0.25;

            throttle_percent_norm = 0.63;

            takeoff_step = takeoff_step + 1;
        end

        if time_sec > 310 && takeoff_step == 18
            manual_trim_time_end = time_sec + 2;
            manual_trim_direction = 1;

            ref_pitch = 0;

            takeoff_step = takeoff_step + 1;
        end

        if time_sec > 315 && takeoff_step == 19
            ref_pitch = 3;

            takeoff_step = takeoff_step + 1;
        end


        if time_sec > 328 && takeoff_step == 20
            flap_cmd_norm = 0;

            throttle_percent_norm = 0.5;

            ref_pitch = -3;

            takeoff_step = takeoff_step + 1;
        end

        if time_sec > 337 && takeoff_step == 21
            manual_trim_time_end = time_sec + 2;
            manual_trim_direction = 1;

            ref_pitch = 7;

            takeoff_step = takeoff_step + 1;
        end

        if time_sec > 350 && takeoff_step == 22

            elevator_mode = elevator_mode_off;

            takeoff_step = takeoff_step + 1;
        end

        if time_sec > 355.3 && takeoff_step == 23

            elevator_mode = elevator_mode_pitch;
            ref_pitch = 4;

            takeoff_step = takeoff_step + 1;
        end

        if time_sec > 356.3 && takeoff_step == 24

            manual_trim_time_end = time_sec + 4;
            manual_trim_direction = 1;

            takeoff_step = takeoff_step + 1;
        end

        if time_sec > 365 && takeoff_step == 25

            throttle_percent_norm = 0.63;

            takeoff_step = takeoff_step + 1;
        end

        if time_sec > 370 && takeoff_step == 26
            
            elevator_mode = elevator_mode_off;

            takeoff_step = takeoff_step + 1;
        end

        if time_sec > 372.3 && takeoff_step == 27

            elevator_mode = elevator_mode_pitch;
            ref_pitch = 2;

            takeoff_step = takeoff_step + 1;
        end

        if time_sec > 376.8 && takeoff_step == 28

            manual_trim_time_end = time_sec + 2.5;
            manual_trim_direction = 1;

            takeoff_step = takeoff_step + 1;
        end

        if time_sec > 380 && takeoff_step == 29

            ref_pitch = -1;

            takeoff_step = takeoff_step + 1;
        end

        if time_sec > 390 && takeoff_step == 30

            elevator_mode = elevator_mode_off;

            throttle_percent_norm = 0.75;

            takeoff_step = takeoff_step + 1;
        end

        if time_sec > 392.8 && takeoff_step == 31

            elevator_mode = elevator_mode_pitch;
            ref_pitch = -5;

            takeoff_step = takeoff_step + 1;
        end

        if time_sec > 395.3 && takeoff_step == 32

            manual_trim_time_end = time_sec + 1;
            manual_trim_direction = 1;

            throttle_percent_norm = 0.63;

            takeoff_step = takeoff_step + 1;
        end

        if time_sec > 398.8 && takeoff_step == 33

            manual_trim_time_end = time_sec + 2;
            manual_trim_direction = 1;

            takeoff_step = takeoff_step + 1;
        end
   
    otherwise
        error("Function block: No valid script selected");
end

%% Output vectors
direct_to_JSBSim = [engine_0_running, engine_1_running, landing_gear_cmd_norm, flap_cmd_norm, left_brake_cmd, right_brake_cmd, param_pilot_reaction];
elevator_sp = [elevator_mode, ref_altitude, ref_vert_speed, ref_pitch, ref_vc, ref_direct];
aileron_sp = [aileron_mode, ref_heading, ref_heading_rate, ref_roll];
rudder_sp = [rudder_mode, ref_beta];
throttle_sp = [throttle_mode, ref_vc, throttle_percent_norm];
horstab_sp = [do_pilot_trim, do_manual_trim, manual_trim_direction];

if isempty(takeoff_stall_retrim_start_time)
    takeoff_stall_retrim_start_time = -999;
end
if isempty(takeoff_stall_last_mcas_turnon_time)
    takeoff_stall_last_mcas_turnon_time = -999;
end
debug = [mcas_is_firing, takeoff_stall_last_mcas_turnon_time];

end % function
